simulink model "act2"  (R2020a)
settings: Solver=ode1  StartTime=0.0  StopTime=10  FixedStep=0.1  RelTol=1e-3
values from neighbouring files (symbols this model uses):
  a_0 = 3    [act2_script.m]
  a_1 = 1    [act1_script.m]    (also in act2_script.m; act3_script.m = 2)
  a_2 = 2    [act1_script.m]    (also in act2_script.m; act3_script.m = 1)
settings Model: Creator=Jorjolo  LastModifiedBy=Jorjolo

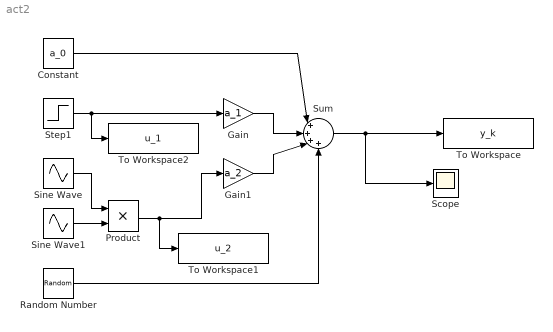
== system act2 ==
  Constant : Constant  Value=a_0
  Gain : Gain  Gain=a_1
  Gain1 : Gain  Gain=a_2
  Product : Product
  Random Number : RandomNumber  Variance=1e-1  SampleTime=0.1
  Scope : Scope
  Sine Wave : Sin  Frequency=10  Samples=100  SampleTime=0
  Sine Wave1 : Sin  Frequency=10  Samples=100  SampleTime=0
  Step1 : Step  SampleTime=0
  Sum : Sum  Inputs=|++++
  To Workspace : ToWorkspace  VariableName=y_k  SampleTime=0.5
  To Workspace1 : ToWorkspace  VariableName=u_2  SampleTime=0.5
  To Workspace2 : ToWorkspace  VariableName=u_1  SampleTime=0.5
  wires:
  Step1/1 -> Gain/1, To Workspace2/1
  Sine Wave/1 -> Product/1
  Sine Wave1/1 -> Product/2
  Product/1 -> To Workspace1/1, Gain1/1
  Gain/1 -> Sum/2
  Constant/1 -> Sum/1
  Random Number/1 -> Sum/4
  Sum/1 -> Scope/1, To Workspace/1
  Gain1/1 -> Sum/3
